simulink library "FCM_lib"  (Simulink 7.4)
settings: Solver=ode45  StartTime=0.0  StopTime=10.0  RelTol=1e-3
values from neighbouring files (symbols this model uses):
  FCMc_c_BCPNomEngy = mpt.Parameter    [FCM_CAL.m]
  FCMc_c_BRMRatCpty = mpt.Parameter    [FCM_CAL.m]
  FCMc_enum_BRMBattType = mpt.Parameter    [FCM_CAL.m]
  FCMc_i_ConstCurReq = mpt.Parameter    [FCM_CAL.m]
  FCMc_i_CurDifThrld = mpt.Parameter    [FCM_CAL.m]
  FCMc_i_CurReq_min = mpt.Parameter    [FCM_CAL.m]
  FCMc_num_BRMProtolVer = mpt.Parameter    [FCM_CAL.m]
  FCMc_t_CellTemp_MaxAlwd = mpt.Parameter    [FCM_CAL.m]
  FCMc_t_CellTemp_MinAlwd = mpt.Parameter    [FCM_CAL.m]
  FCMc_tm_ConstVoltTime = mpt.Parameter    [FCM_CAL.m]
  FCMc_tm_FastEndCondt = mpt.Parameter    [FCM_CAL.m]
  FCMc_v_BRMPackRatVolt = mpt.Parameter    [FCM_CAL.m]
  FCMc_v_VoltDifThrld = mpt.Parameter    [FCM_CAL.m]
  FCMm_c_CellChaC_AH = mpt.Parameter    [FCM_CAL.m]
  FCMm_i_CurrArrayT = mpt.Parameter    [FCM_CAL.m]
  FCMx_t_CelltempArrayT = mpt.Parameter    [FCM_CAL.m]
undefined symbols (not defined in the file or in its folder): BATc_pct_PackSocAlwd, BATc_v_CellVolt_MaxAlwd, BATc_v_CellVolt_MinAlwd, BATc_v_ConstVoltCell, BATc_v_PackVoltAlwd, FCM_Charging_St, PACK_Const_ParaCellNumOfMdl
libraries: Defined_Functionality x18
(part 2 of 2)

== stateflow chart FCM/FCM_BCL/debounce1/debounce ==
  state No_Debounce
    No_Debounce -> (junction 11) [order 1]
    (default) -> (junction 11)
    (junction 11) -> (junction 10) : {out=in;}
  state Debounce
    state TURE
      out=1;
    state Wait
      state To_on
        To_on -> (junction 15) [order 1]
        (junction 15) -> (junction 13) : {Timer_On++;}
        (default) -> (junction 15) : {Timer_On=1;}
      state To_off
        To_off -> (junction 12) [order 1]
        (junction 12) -> (junction 17) : {Timer_Off++;}
        (default) -> (junction 12) : {Timer_Off=1;}
    state FALSE
      out=0;
    FALSE -> To_on [order 2] : [in==1]
    To_off -> TURE [order 1] : [in==1]
    TURE -> To_off : [in==0]
    (junction 14) -> FALSE
    To_on -> (junction 16) [order 1] : [10*Timer_On>=debounce_time&&in!=0]
    (junction 16) -> TURE
    To_off -> (junction 14) [order 2] : [10*Timer_Off>=debounce_time&&in!=1]
    To_on -> FALSE [order 2] : [in==0]
    (default) -> FALSE
  (default) -> Debounce
  FALSE -> No_Debounce [order 1] : [debounce_time==0]
  No_Debounce -> FALSE [order 1] : [debounce_time!=0]
  data: in input boolean; out output boolean; count_timer local uint32; Timer_Off local uint32; Timer_On local uint32; debounce_time parameter uint32

== stateflow chart FCM/FCM_FLOW ==
  state FCM_NoChage
    en:
    FCMd_enum_ChaSt = FCM_NoCharge_St;
    FCMd_enum_BEMTimeOver3901 = 0;
    FCMd_enum_BEMTimeOver3902 = 0;
    FCMd_enum_BEMTimeOver3903 = 0;
    FCMd_enum_BEMTimeOver3904 = 0;
    settings: description=$Author:Zhao XiangRi$
  state FCM_Finished
    state FCM_Finished_BSD
      en:
      FCMd_flg_BSDTM = 1;
      du:
      Timer.T2.Run(FCMc_tm_FinishDly);
      ex:
      Timer.T1.Clear();
      FCMd_flg_BSDTM = 0;
    state FCM_Finished_Init
      en:
      FCMd_enum_ChaSt =FCM_ChaFinished_St;
      FCMd_flg_BSTTM = 1;
      du:
      Timer.T1.Run(FCMc_tm_FinishDly);
      ex:
      Timer.T1.Clear();
      FCMd_flg_BSTTM = 0;
    state FCM_Finished_BEM
      en:
      FCMd_flg_BEMTM = 1;
      FCMd_enum_ChaSt = FCM_ChaTimeOver_St;
      FCMd_enum_ChaCtrCmd = CTC_FastChaOffline_CtrCmd;
      ex:
      FCMd_flg_BEMTM = 0;
    state FCM_Finished_Exit
      en:
      FCMd_enum_ChaCtrCmd = CTC_FastChaOffline_CtrCmd;
    FCM_Finished_Init -> FCM_Finished_BSD [order 1] : [IPTd_flg_CSTRX == 1 ...
        |  && Timer.T1.Timeout1  != 1 ]
    (junction 79) -> FCM_Finished_BEM : {FCMd_enum_BEMTimeOver3906 = 1;}
    FCM_Finished_Init -> (junction 79) [order 2] : [Timer.T1.Timeout1  == 1]
    (default) -> FCM_Finished_Init
    (junction 78) -> FCM_Finished_BEM : {FCMd_enum_BEMTimeOver3907 = 1;}
    FCM_Finished_BSD -> FCM_Finished_Exit [order 1] : [IPTd_flg_CSDRX == 1 ...
        | &&Timer.T2.Timeout2 != 1]
    FCM_Finished_BSD -> (junction 78) [order 2] : [Timer.T2.Timeout2 == 1]
  state FCM_Charging
    ex:
    FCMd_flg_BCLTM  = 0;
    FCMd_flg_BCSTM = 0;
    state FCM_Charging_BSM
      en:
      FCMd_flg_BSMTM = 1;
      FCMd_flg_BMVTM = 1;
      FCMd_flg_BMTTM = 1;
      ex:
      FCMd_flg_BSMTM = 0;
      FCMd_flg_BMVTM = 0;
      FCMd_flg_BMTTM = 0;
    state FCM_Charging_BEM
      en:
      FCMd_enum_ChaSt = FCM_ChaTimeOver_St ;
      FCMd_flg_BEMTM = 1;
      ex:
      FCMd_flg_BEMTM = 0;
    state FCM_Charging_BCL
      en:
      FCMd_enum_ChaSt = FCM_Charging_St;
      FCMd_flg_BCLTM  = 1;
      FCMd_flg_BCSTM = 1;
      du:
      Timer.T1.Run(FCMc_tm_ChaDly);
      ex:
      Timer.T1.Clear();
    (junction 86) -> (junction 84) : [FCMd_flg_BSMChaAlwd == 1 ...
        | && IPTd_flg_CSTRX == 0]
    FCM_Charging_BSM -> (junction 86)
    FCM_Charging_BCL -> FCM_Charging_BSM [order 1] : [IPTd_flg_CCSRX == 1 ...
        | && Timer.T1.Timeout1 != 1]
    (junction 80) -> FCM_Charging_BEM : {FCMd_enum_BEMTimeOver3905 = 1;...
        | FCMd_flg_BCLTM  = 0;...
        | FCMd_flg_BCSTM = 0;}
    (junction 84) -> (junction 81)
    FCM_Charging_BCL -> (junction 80) [order 2] : [Timer.T1.Timeout1  == 1]%the times  to be 100ms
    (junction 81) -> FCM_Charging_BCL
    (default) -> FCM_Charging_BCL
  state FCM_HandShaking
    state FCM_HandsShake_Init
      en:
      FCMd_enum_ChaSt = FCM_Handshaking_St;
      du:
      Timer.T1.Run(FCMc_tm_ShakeDly);
      ex:
      Timer.T1.Clear();
    state FCM_HandShake_BEM
      en:
      FCMd_enum_ChaSt = FCM_ChaTimeOver_St;
      FCMd_flg_BEMTM = 1;
      ex:
      FCMd_flg_BEMTM = 0;
    state FCM_HandShake_BRM
      en:
      FCMd_flg_BRMTM = 1;
      du:
      Timer.T2.Run(FCMc_tm_ShakeDly);
      ex:
      Timer.T2.Clear();
      FCMd_flg_BRMTM = 0;
    (default) -> FCM_HandsShake_Init
    FCM_HandsShake_Init -> (junction 92) [order 1] : [Timer.T1.Timeout1  == 1 ]%the times to be 5S
    (junction 92) -> FCM_HandShake_BEM : {FCMd_enum_BEMTimeOver3901 = 1;}
    FCM_HandsShake_Init -> FCM_HandShake_BRM [order 2] : [IPTd_flg_CRMRX == true&&...
        | Timer.T1.Timeout1 != 1&&...
        | IPTd_enum_CRMRecgResult == 0]
    FCM_HandShake_BRM -> (junction 95) : [Timer.T2.Timeout2  == 1]
    (junction 95) -> FCM_HandShake_BEM : {FCMd_enum_BEMTimeOver3902 = 1;}
  state FCM_ParametesConfiguration
    state FCM_Config_Exit
      du:
      FCMd_enum_ChaCtrCmd = CTC_FastChaOnline_CtrCmd;
    state FCM_Config_BCP
      en:
      FCMd_enum_ChaSt = FCM_Configuration_St;
      FCMd_flg_BCPTM = 1;
      du:
      Timer.T1.Run(FCMc_tm_ConfigDly);
      ex:
      Timer.T1.Clear();
      FCMd_flg_BCPTM = 0;
    state FCM_Config_BROExit
      en:
      FCMd_flg_BROTM = 1;
      FCMd_enum_BROBattChaReady = 0;
      FCMd_enum_ChaSt = FCM_ChaTimeOver_St;
      ex:
      FCMd_flg_BROTM = 0;
    state FCM_Config_BROIn
      en:
      FCMd_enum_BROBattChaReady = 170;
      FCMd_flg_BROTM = 1;
      du:
      Timer.T2.Run(FCMc_tm_ConfigDly);
      ex:
      Timer.T2.Clear();
      FCMd_flg_BROTM = 0;
    state FCM_Config_BEM
      en:
      FCMd_flg_BEMTM = 1;
      FCMd_enum_ChaSt = FCM_ChaTimeOver_St;
      ex:
      FCMd_flg_BEMTM = 0;
    (default) -> FCM_Config_BCP
    FCM_Config_BCP -> (junction 89) [order 2] : [Timer.T1.Timeout1  == 1]
    (junction 89) -> FCM_Config_BEM : {FCMd_enum_BEMTimeOver3903 = 1;}
    FCM_Config_BCP -> (junction 88) [order 1] : [IPTd_flg_CTSRX == 1 ...
        |  && IPTd_flg_CMLRX == 1 ...
        |  && Timer.T1.Timeout1  != 1]%need cts and cms both receive
    (junction 85) -> FCM_Config_BEM : {FCMd_enum_BEMTimeOver3904 = 1;}
    (junction 88) -> FCM_Config_BROExit [order 2] : [FCMd_flg_BSMChaAlwd == 0]
    (junction 88) -> FCM_Config_BROIn [order 1] : [FCMd_flg_BSMChaAlwd == 1]
    FCM_Config_BROIn -> (junction 85) [order 2] : [ Timer.T2.Timeout2  == 1]%the times  to be 5S
    (junction 83) -> FCM_Config_BROIn
    FCM_Config_BROIn -> (junction 82) [order 1] : [IPTd_flg_CRORX == 1 ...
        |  && Timer.T2.Timeout2  != 1]
    (junction 82) -> (junction 83) [order 2] : [IPTd_enum_CROChagrOptReady == 0 ...
        |  || IPTd_enum_CROChagrOptReady == 255]
    (junction 82) -> FCM_Config_Exit [order 1] : [IPTd_enum_CROChagrOptReady == 170]
  state Timer [function]
    state T1 [function]
      settings: description=$Author:Zhao XiangRi$
      state Run(Limit1) [function]
        settings: description=$Author:Zhao XiangRi$
        (default) -> (junction 96)
        (junction 96) -> (junction 97) [order 1] : [Init1 != 1]
            | {TimeTicks1 = 0;TimeLimit1 = Limit1/10;Init1 = 1;}
        (junction 97) -> (junction 96)
        (junction 96) -> (junction 98) [order 2] : {TimeTicks1++;}
        (junction 98) -> (junction 99) [order 1] : [TimeTicks1 >= TimeLimit1]{Timeout1 = 1;}
        (junction 98) -> (junction 100) [order 2]
      state Clear [function]
        settings: description=$Author:Zhao XiangRi$
        (default) -> (junction 101)
        (junction 101) -> (junction 102) : {Timeout1 = 0;Init1 = 0;}
    state T2 [function]
      settings: description=$Author:Zhao XiangRi$
      state Run(Limit2) [function]
        settings: description=$Author:Zhao XiangRi$
        (default) -> (junction 103)
        (junction 103) -> (junction 104) [order 1] : [Init2 != 1]{TimeTicks2 = 0;TimeLimit2 = Limit2/10 ;Init2 = 1;}
        (junction 104) -> (junction 103)
        (junction 103) -> (junction 105) [order 2] : {TimeTicks2++;}
        (junction 105) -> (junction 106) [order 1] : [TimeTicks2 >= TimeLimit2]{Timeout2 = 1;}
        (junction 105) -> (junction 107) [order 2]
      state Clear [function]
        settings: description=$Author:Zhao XiangRi$
        (default) -> (junction 108)
        (junction 108) -> (junction 109) : {Timeout2 = 0;
            | Init2 = 0;}
  (junction 93) -> (junction 94)
  (junction 90) -> (junction 91)
  (default) -> FCM_NoChage
  FCM_HandShaking -> FCM_ParametesConfiguration [order 2] : [IPTd_flg_CRMRX == 1&&...
      | IPTd_enum_CRMRecgResult== 170]
  FCM_Charging -> FCM_Finished [order 2] : [FCMd_flg_BSMChaAlwd == 0 ...
      | || (IPTd_flg_CSTRX == 1&&FCMd_flg_CSTChaStop==1)]
  FCM_ParametesConfiguration -> FCM_Charging [order 2] : [CTCd_enum_CtrSt==CTC_FastChaOnline_St ...
      | &&FCMd_enum_ChaCtrCmd == CTC_FastChaOnline_CtrCmd]
  FCM_ParametesConfiguration -> (junction 90) [order 1] : [FCMd_enum_ChaSt == FCM_ChaTimeOver_St]
  FCM_HandShaking -> (junction 91) [order 1] : [FCMd_enum_ChaSt == FCM_ChaTimeOver_St]
  (junction 94) -> FCM_Finished
  (junction 87) -> FCM_NoChage
  FCM_Charging -> (junction 93) [order 1] : [FCMd_enum_ChaSt == FCM_ChaTimeOver_St]
      | {FCMd_enum_BEMTimeOver3905 = 0;}
  FCM_NoChage -> FCM_HandShaking : [BSCd_enum_BCUSt==BCU_FastCharge_St]
  (junction 91) -> (junction 87)
  data: Timeout1 local boolean; TimeLimit1 local single; Init1 local boolean; TimeTicks1 local single; Limit1 function_input single; Timeout2 local boolean; TimeLimit2 local single; TimeTicks2 local single; Init2 local boolean; Limit2 function_input single; FCMd_flg_CSTChaStop input double; BCU_FastCharge_St parameter uint8; CTC_FastChaOnline_CtrCmd parameter uint8; CTC_FastChaOnline_St parameter uint8; CTC_FastChaOffline_CtrCmd parameter uint8; BSCd_enum_BCUSt input uint8; IPTd_enum_CRMRecgResult input double; IPTd_enum_CROChagrOptReady input double; CTCd_enum_CtrSt input uint8; FCMd_flg_BSMChaAlwd input boolean; FCM_NoCharge_St parameter uint8; FCM_Handshaking_St parameter uint8; FCM_Configuration_St parameter uint8; FCM_Charging_St parameter uint8; FCM_ChaFinished_St parameter uint8; FCM_ChaTimeOver_St parameter uint8; IPTd_flg_CCSRX input boolean; IPTd_flg_CMLRX input boolean; IPTd_flg_CRORX input boolean; IPTd_flg_CSDRX input boolean; IPTd_flg_CSTRX input boolean; IPTd_flg_CTSRX input boolean; IPTd_flg_CRMRX input boolean; FCMd_enum_BEMTimeOver3901 output uint8; FCMd_enum_BEMTimeOver3902 output uint8; FCMd_enum_BEMTimeOver3903 output uint8; FCMd_enum_BEMTimeOver3904 output uint8; FCMd_enum_BEMTimeOver3905 output uint8; FCMd_enum_BEMTimeOver3906 output uint8; FCMd_enum_BEMTimeOver3907 output uint8; FCMd_flg_BRMTM output boolean; FCMd_flg_BCPTM output boolean; FCMd_flg_BROTM output boolean; FCMd_flg_BCLTM output boolean; FCMd_flg_BCSTM output boolean; FCMd_flg_BSMTM output boolean; FCMd_flg_BMVTM output boolean; FCMd_flg_BMTTM output boolean; FCMd_flg_BSTTM output boolean; FCMd_flg_BSDTM output boolean; FCMd_flg_BEMTM output boolean; FCMd_enum_ChaCtrCmd output uint8; FCMd_enum_BROBattChaReady output uint8; FCMd_enum_ChaSt output uint8; FCMc_tm_ShakeDly parameter uint16; FCMc_tm_ConfigDly parameter uint16; FCMc_tm_ChaDly parameter uint16; FCMc_tm_FinishDly parameter uint16

== stateflow chart FCM/FCM_BCL/FCM_BCL ==
  state Timer [function]
    state T1 [function]
      settings: description=$Author:Zhao XiangRi$
      state Run(Limit1) [function]
        settings: description=$Author:Zhao XiangRi$
        (default) -> (junction 243)
        (junction 243) -> (junction 244) [order 1] : [Init1 != 1]
            | {TimeTicks1 = 0;TimeLimit1 = Limit1/10;Init1 = 1;}
        (junction 244) -> (junction 243)
        (junction 243) -> (junction 245) [order 2] : {TimeTicks1++;}
        (junction 245) -> (junction 246) [order 1] : [TimeTicks1 >= TimeLimit1]{Timeout1 = 1;}
        (junction 245) -> (junction 247) [order 2]
      state Clear [function]
        settings: description=$Author:Zhao XiangRi$
        (default) -> (junction 248)
        (junction 248) -> (junction 249) : {Timeout1 = 0;Init1 = 0;}
  state FCM_ConstCurCharging
    state FCM_Init
      en:
      FCMd_flg_ChaStopReq = false;
      FCMd_i_CurReq = FCMc_i_CurReq_min;
      FCMd_i_BCLBattChaCurReq = - FCMd_i_CurReq ;
      FCMd_mode_BCLBattChaReq = ConstCurrChaMode;
      FCMd_v_BCLBattChaVoltReq=FCMd_v_PackChaVoltMax;
    state FCM_Curr_Addcout
      du:Timer.T1.Run(FCMc_tm_CurAddDly);
    state FCM_Curr_AddStep
      en:
      FCMd_i_BCLBattChaCurReq = -FCMd_i_CurReq;
      FCMd_i_CurReq+=FCMc_i_CurReq_min;
      Timer.T1.Clear();
    state FCM_Curr_Const
      en:
      FCMd_i_BCLBattChaCurReq = -FCMd_i_ConstCurReq;
      du:
      FCMd_i_BCLBattChaCurReq = -FCMd_i_ConstCurReq;
    (default) -> FCM_Init
    FCM_Init -> FCM_Curr_Addcout
    (junction 250) -> FCM_Curr_Addcout
    (junction 251) -> (junction 250)
    FCM_Curr_Addcout -> FCM_Curr_AddStep : [Timer.T1.Timeout1 == 1]
    FCM_Curr_AddStep -> (junction 251) [order 2] : [FCMd_i_ShuntCurAbs < FCMd_i_ConstCurReq&&...
        | FCMd_i_CurReq<FCMd_i_ConstCurReq]
    FCM_Curr_AddStep -> FCM_Curr_Const [order 1] : [FCMd_i_CurReq>=FCMd_i_ConstCurReq]
  state FCM_ConstVoltCharging
    en:
    FCMd_mode_BCLBattChaReq = ConstVoltChaMode;
    FCMd_v_BCLBattChaVoltReq=IPTd_v_PosCtrVoltRef1_front;
    FCMd_i_BCLBattChaCurReq = -FCMd_i_ConstCurReq;
  state FCM_ChaFinished
    en:
    FCMd_flg_ChaStopReq = true;
  FCM_ConstCurCharging -> FCM_ConstVoltCharging : [FCMd_flg_ConstVoltCharging == 1]
  FCM_ConstVoltCharging -> FCM_ChaFinished : [FCMd_flg_FastChaStop==1]
  (default) -> FCM_ConstCurCharging
  data: Timeout1 local boolean; TimeLimit1 local single; TimeTicks1 local single; Init1 local boolean; Limit1 function_input single; FCMd_v_BCLBattChaVoltReq output single; FCMc_i_CurReqStep parameter single; FCMc_tm_CurAddDly parameter single; FCMd_i_ConstCurReq input single; IPTd_v_CellVolt_max input single; FCMd_i_BCLBattChaCurReq output single; FCMd_mode_BCLBattChaReq output uint8; FCMd_flg_ConstVoltCharging input boolean; IPTd_v_PosCtrVoltRef1_front input double; FCMd_flg_FastChaStop input boolean; FCMc_v_CellVoltDelta parameter single; FCMc_v_PackVoltDelta parameter single; FCMd_flg_ChaStopReq output boolean; ConstCurrChaMode parameter uint8; ConstVoltChaMode parameter uint8; FCMc_i_CurReq_min parameter single; FCMd_i_CurReq local single; FCMd_i_ShuntCurAbs input double; FCMd_v_PackChaVoltMax parameter double
